simulink model "gm_smartCart4_1_work"  (R2016a)
settings: Solver=FixedStepDiscrete  StartTime=0.0  StopTime=100000  FixedStep=1  RelTol=1e-3
libraries: simulink x103, hdlsllib x73
(part 1 of 3)
settings Model: Creator=Admin  LastModifiedBy=Admin
settings OptimizationCC: BlockReduction=off  ConditionallyExecuteInputs=off  DefaultParameterBehavior=Inlined
settings DebuggingCC: AlgebraicLoopMsg=error  InheritedTsInSrcMsg=none
settings HardwareCC: ProdBitPerPointer=32  ProdLargestAtomicFloat=None  ProdIntDivRoundTo=Undefined  ProdEndianess=Unspecified  ProdWordSize=32  ProdHWDeviceType=ASIC/FPGA->ASIC/FPGA  ProdEqTarget=off

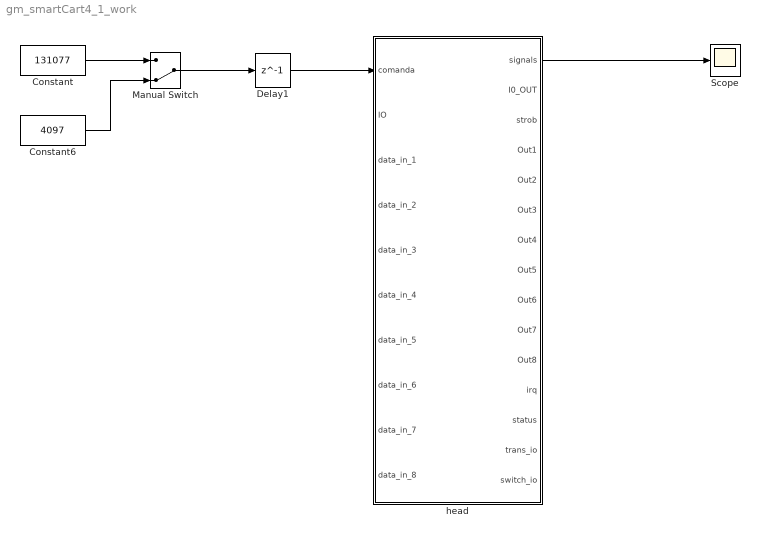
== system gm_smartCart4_1_work ==
  Constant : Constant  Value=131077  OutDataTypeStr=uint32  SampleTime=-1
  Constant6 : Constant  Value=4097  OutDataTypeStr=uint32  SampleTime=-1
  Delay1 : Delay  DelayLength=1  InitialCondition=0
  Manual Switch : ManualSwitch  CurrentSetting=0
  Scope : Scope
  head : Subsystem  TreatAsAtomicUnit=on
  wires:
  head/1(signals) -> Scope/1
  Delay1/1 -> head/1(comanda)
  Manual Switch/1 -> Delay1/1
  Constant6/1 -> Manual Switch/2
  Constant/1 -> Manual Switch/1

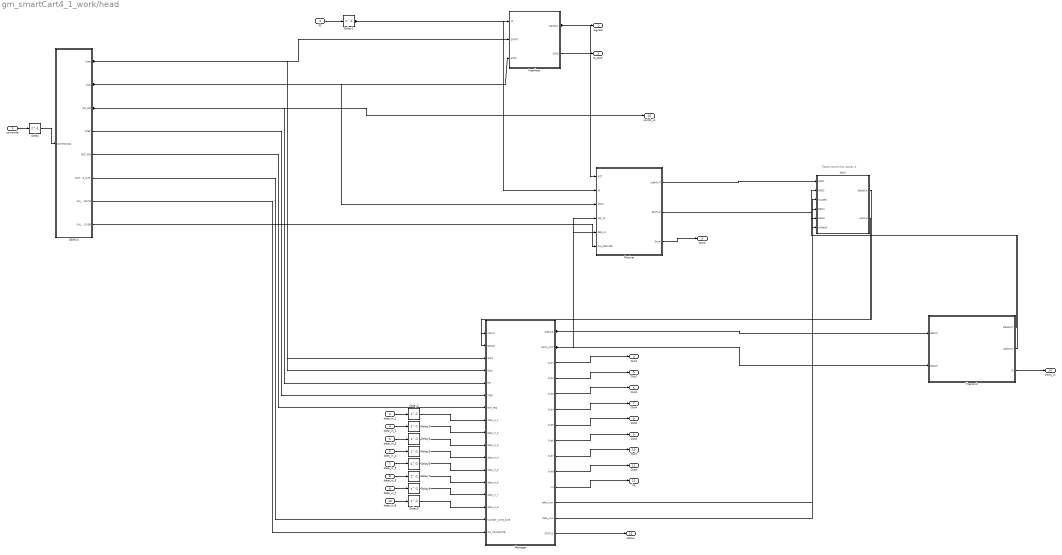
== system gm_smartCart4_1_work/head ==
  note: Переключатель адрес 4
  comanda : Inport  OutDataTypeStr=uint32  SampleTime=1
  IO : Inport  Port=2  OutDataTypeStr=boolean
  data_in_1 : Inport  Port=3  OutDataTypeStr=uint32
  data_in_2 : Inport  Port=4  OutDataTypeStr=uint32
  data_in_3 : Inport  Port=5  OutDataTypeStr=uint32
  data_in_4 : Inport  Port=6  OutDataTypeStr=uint32
  data_in_5 : Inport  Port=7  OutDataTypeStr=uint32
  data_in_6 : Inport  Port=8  OutDataTypeStr=uint32
  data_in_7 : Inport  Port=9  OutDataTypeStr=uint32
  data_in_8 : Inport  Port=10  OutDataTypeStr=uint32
  DEMUX : Subsystem
  Delay{,1..9} (10 alike) : Delay  DelayLength=1  InitialCondition=0
  Interface : Subsystem
  MUX : Subsystem
  Manager : Subsystem
  Reciver : Subsystem
  Transmit : Subsystem
  signals : Outport  OutDataTypeStr=fixdt(1,4,0)
  I0_OUT : Outport  Port=2  OutDataTypeStr=boolean
  strob : Outport  Port=3  OutDataTypeStr=boolean
  Out1 : Outport  Port=4  OutDataTypeStr=uint8
  Out2 : Outport  Port=5  OutDataTypeStr=uint8
  Out3 : Outport  Port=6  OutDataTypeStr=uint8
  Out4 : Outport  Port=7  OutDataTypeStr=uint8
  Out5 : Outport  Port=8  OutDataTypeStr=uint8
  Out6 : Outport  Port=9  OutDataTypeStr=uint8
  Out7 : Outport  Port=10  OutDataTypeStr=uint8
  Out8 : Outport  Port=11  OutDataTypeStr=uint8
  irq : Outport  Port=12  OutDataTypeStr=boolean
  status : Outport  Port=13  OutDataTypeStr=uint32
  trans_io : Outport  Port=14  OutDataTypeStr=boolean
  switch_io : Outport  Port=15  OutDataTypeStr=boolean
  wires:
  comanda/1 -> Delay/1
  IO/1 -> Delay1/1
  data_in_1/1 -> Delay2/1
  data_in_2/1 -> Delay3/1
  data_in_3/1 -> Delay4/1
  data_in_4/1 -> Delay5/1
  data_in_5/1 -> Delay6/1
  data_in_6/1 -> Delay7/1
  data_in_7/1 -> Delay8/1
  data_in_8/1 -> Delay9/1
  DEMUX/1(start) -> Interface/2(START), Manager/3(Start)
  DEMUX/2(stop) -> Interface/3(STOP), Reciver/3(STOP), Manager/4(Stop)
  DEMUX/3(RD_WR) -> Manager/5(RD), switch_io/1
  DEMUX/4(STEP) -> Manager/6(STEP)
  DEMUX/5(RST_IRQ) -> Manager/7(RST_IRQ)
  DEMUX/6(Number_write_byte) -> Manager/16(Number_write_byte)
  DEMUX/7(ON_TRANSMITE) -> Manager/17(ON_TRANSMITE)
  DEMUX/8(ON_RECIVER) -> Reciver/6(ON_RECIVER)
  Delay/1 -> DEMUX/1(COMMANDA)
  Delay1/1 -> Reciver/2(IO), Interface/1(IO)
  Delay2/1 -> Manager/8(data_in_1)
  Delay3/1 -> Manager/9(data_in_2)
  Delay4/1 -> Manager/10(data_in_3)
  Delay5/1 -> Manager/11(data_in_4)
  Delay6/1 -> Manager/12(data_in_5)
  Delay7/1 -> Manager/13(data_in_6)
  Delay8/1 -> Manager/14(data_in_7)
  Delay9/1 -> Manager/15(data_in_8)
  Interface/1(signals2) -> Reciver/1(RST), signals/1
  Interface/2(Out3) -> I0_OUT/1
  MUX/1(DataOut) -> Manager/2(DataIN)
  MUX/2(AdrOut) -> Manager/1(AdrrIN)
  Manager/1(addrout) -> Transmit/1(addrIN), Reciver/4(adr_IN)
  Manager/2(DATA_OUT) -> Transmit/2(dataIN), Reciver/5(data_in)
  Manager/3(Out1) -> Out1/1
  Manager/4(Out2) -> Out2/1
  Manager/5(Out3) -> Out3/1
  Manager/6(Out4) -> Out4/1
  Manager/7(Out5) -> Out5/1
  Manager/8(Out6) -> Out6/1
  Manager/9(Out7) -> Out7/1
  Manager/10(Out8) -> Out8/1
  Manager/11(irq) -> irq/1
  Manager/12(addr_mux) -> MUX/3(mADR3)
  Manager/13(data_mux) -> MUX/6(mData3)
  Manager/14(STATUS) -> status/1
  Reciver/1(AddrOUT) -> MUX/1(ADR1)
  Reciver/2(STATUS) -> MUX/4(Data1)
  Reciver/3(Strob) -> strob/1
  Transmit/1(DataOUT) -> MUX/5(Data2)
  Transmit/2(addrOUT) -> MUX/2(ADR2)
  Transmit/3(IO) -> trans_io/1

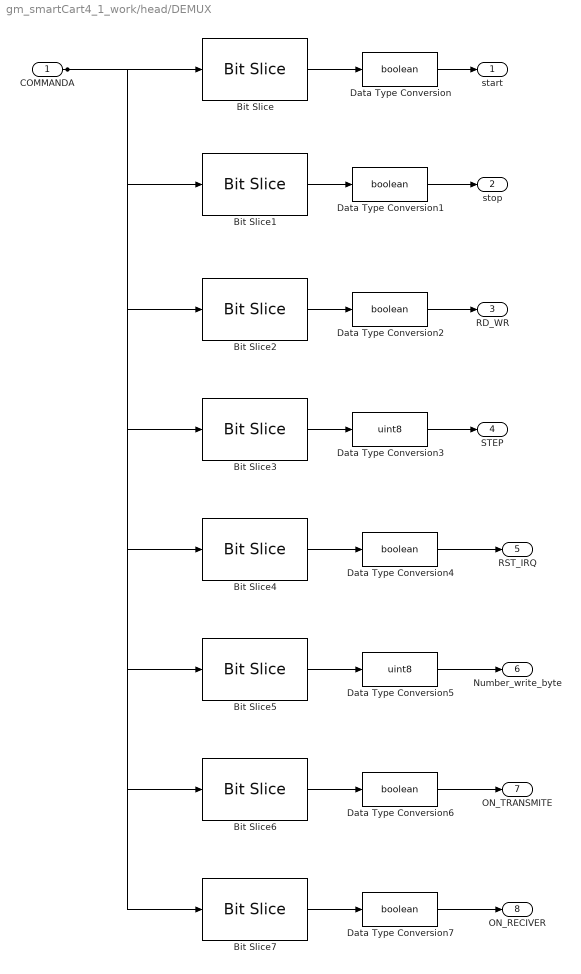
== system gm_smartCart4_1_work/head/DEMUX ==
  COMMANDA : Inport  OutDataTypeStr=uint32  SampleTime=1
  Bit Slice : hdlsllib/HDL Operations/Bit Slice  lidx=0  ridx=0
  Bit Slice1 : hdlsllib/HDL Operations/Bit Slice  lidx=1  ridx=1
  Bit Slice2 : hdlsllib/HDL Operations/Bit Slice  lidx=2  ridx=2
  Bit Slice3 : hdlsllib/HDL Operations/Bit Slice  lidx=11  ridx=3
  Bit Slice4 : hdlsllib/HDL Operations/Bit Slice  lidx=12  ridx=12
  Bit Slice5 : hdlsllib/HDL Operations/Bit Slice  lidx=15  ridx=13
  Bit Slice6 : hdlsllib/HDL Operations/Bit Slice  lidx=16  ridx=16
  Bit Slice7 : hdlsllib/HDL Operations/Bit Slice  lidx=17  ridx=17
  Data Type Conversion{,1..2,4,6..7} (6 alike) : DataTypeConversion  OutDataTypeStr=boolean
  Data Type Conversion3 : DataTypeConversion  OutDataTypeStr=uint8
  Data Type Conversion5 : DataTypeConversion  OutDataTypeStr=uint8
  start : Outport
  stop : Outport  Port=2
  RD_WR : Outport  Port=3
  STEP : Outport  Port=4  OutDataTypeStr=uint8
  RST_IRQ : Outport  Port=5
  Number_write_byte : Outport  Port=6  OutDataTypeStr=uint8
  ON_TRANSMITE : Outport  Port=7  OutDataTypeStr=boolean
  ON_RECIVER : Outport  Port=8  OutDataTypeStr=boolean
  wires:
  COMMANDA/1 -> Bit Slice7/1, Bit Slice6/1, Bit Slice5/1, Bit Slice4/1, Bit Slice3/1, Bit Slice2/1, Bit Slice1/1, Bit Slice/1
  Bit Slice/1 -> Data Type Conversion/1
  Bit Slice1/1 -> Data Type Conversion1/1
  Bit Slice2/1 -> Data Type Conversion2/1
  Bit Slice3/1 -> Data Type Conversion3/1
  Bit Slice4/1 -> Data Type Conversion4/1
  Bit Slice5/1 -> Data Type Conversion5/1
  Bit Slice6/1 -> Data Type Conversion6/1
  Bit Slice7/1 -> Data Type Conversion7/1
  Data Type Conversion/1 -> start/1
  Data Type Conversion1/1 -> stop/1
  Data Type Conversion2/1 -> RD_WR/1
  Data Type Conversion3/1 -> STEP/1
  Data Type Conversion4/1 -> RST_IRQ/1
  Data Type Conversion5/1 -> Number_write_byte/1
  Data Type Conversion6/1 -> ON_TRANSMITE/1
  Data Type Conversion7/1 -> ON_RECIVER/1

== system gm_smartCart4_1_work/head/Interface ==
  IO : Inport  OutDataTypeStr=boolean  SampleTime=1
  START : Inport  Port=2  OutDataTypeStr=boolean  SampleTime=1
  STOP : Inport  Port=3  OutDataTypeStr=boolean  SampleTime=1
  ColdStart : Subsystem
  ColdStop2 : Subsystem
  Head2 : Subsystem
  MUX2 : Subsystem
  Swith_signal2 : Subsystem
  signals2 : Outport  OutDataTypeStr=fixdt(1,4,0)  InitialOutput=0
  Out3 : Outport  Port=2  OutDataTypeStr=boolean  InitialOutput=0
  wires:
  IO/1 -> Out3/1, ColdStart/1(Reqest)
  START/1 -> Head2/3(START)
  STOP/1 -> Head2/4(STOP)
  ColdStart/1(DataOUT) -> MUX2/5(DAT_ST1)
  ColdStart/2(Signal) -> MUX2/2(DATA_0)
  ColdStart/3(ADR_OUT) -> MUX2/4(ADR_ST)
  ColdStop2/1(DataOUT) -> MUX2/7(DAT_STOP)
  ColdStop2/2(Signal) -> MUX2/3(DATA_1)
  ColdStop2/3(ADR_OUT) -> MUX2/6(ADR_STOP)
  Head2/1(AdrOut) -> Swith_signal2/1(Adr), ColdStart/2(Addr), ColdStop2/1(Addr)
  Head2/2(DataOut) -> Swith_signal2/2(Data), ColdStart/3(Data), ColdStop2/2(Data)
  MUX2/1(Signals) -> signals2/1
  MUX2/2(ADR_OUT) -> Head2/1(ADR_IN)
  MUX2/3(DATA_OUT1) -> Head2/2(DataIN)
  Swith_signal2/1(OutAddr) -> MUX2/1(ADR)

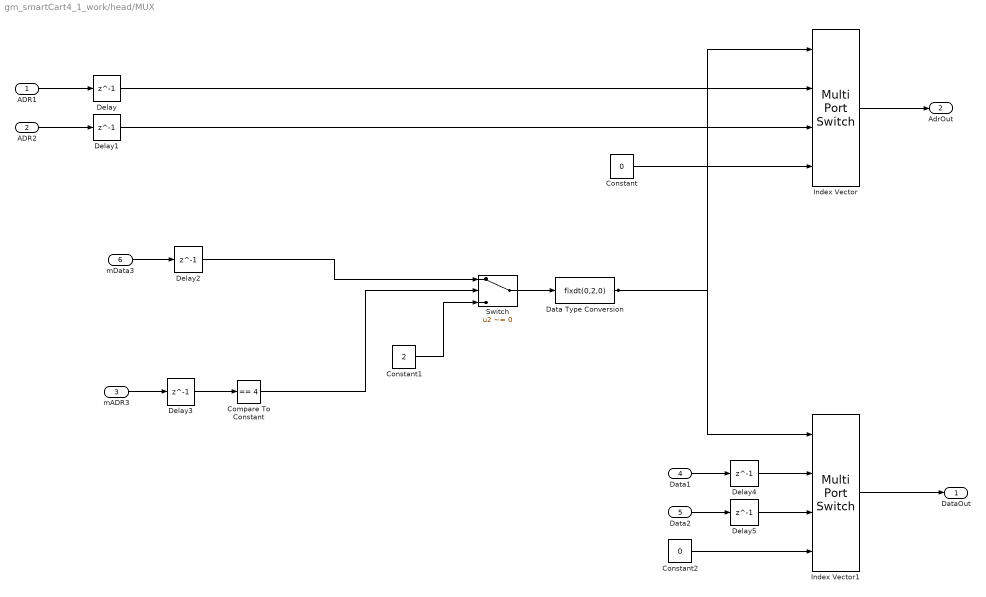
== system gm_smartCart4_1_work/head/MUX ==
  ADR1 : Inport  OutDataTypeStr=uint8  SampleTime=1
  ADR2 : Inport  Port=2  OutDataTypeStr=uint8  SampleTime=1
  mADR3 : Inport  Port=3  OutDataTypeStr=uint8  SampleTime=1
  Data1 : Inport  Port=4  OutDataTypeStr=uint32  SampleTime=1
  Data2 : Inport  Port=5  OutDataTypeStr=uint32  SampleTime=1
  mData3 : Inport  Port=6  OutDataTypeStr=uint32  SampleTime=1
  Compare To Constant : simulink/Logic and Bit Operations/Compare To Constant  relop===  const=4  OutDataTypeStr=boolean
  Constant : Constant  Value=0  OutDataTypeStr=uint8
  Constant1 : Constant  Value=2  OutDataTypeStr=uint32
  Constant2 : Constant  Value=0  OutDataTypeStr=uint32
  Data Type Conversion : DataTypeConversion  OutDataTypeStr=fixdt(0,2,0)
  Delay{,1..5} (6 alike) : Delay  DelayLength=1  InitialCondition=0
  Index Vector : MultiPortSwitch  DataPortOrder=Zero-based contiguous  zeroidx=on
  Index Vector1 : MultiPortSwitch  DataPortOrder=Zero-based contiguous  zeroidx=on
  Switch : Switch  Criteria=u2 ~= 0
  DataOut : Outport  OutDataTypeStr=uint32
  AdrOut : Outport  Port=2  OutDataTypeStr=uint8
  wires:
  ADR1/1 -> Delay/1
  ADR2/1 -> Delay1/1
  mADR3/1 -> Delay3/1
  Data1/1 -> Delay4/1
  Data2/1 -> Delay5/1
  mData3/1 -> Delay2/1
  Compare To Constant/1 -> Switch/2
  Constant/1 -> Index Vector/4
  Constant1/1 -> Switch/3
  Constant2/1 -> Index Vector1/4
  Data Type Conversion/1 -> Index Vector1/1, Index Vector/1
  Delay/1 -> Index Vector/2
  Delay1/1 -> Index Vector/3
  Delay2/1 -> Switch/1
  Delay3/1 -> Compare To Constant/1
  Delay4/1 -> Index Vector1/2
  Delay5/1 -> Index Vector1/3
  Index Vector/1 -> AdrOut/1
  Index Vector1/1 -> DataOut/1
  Switch/1 -> Data Type Conversion/1

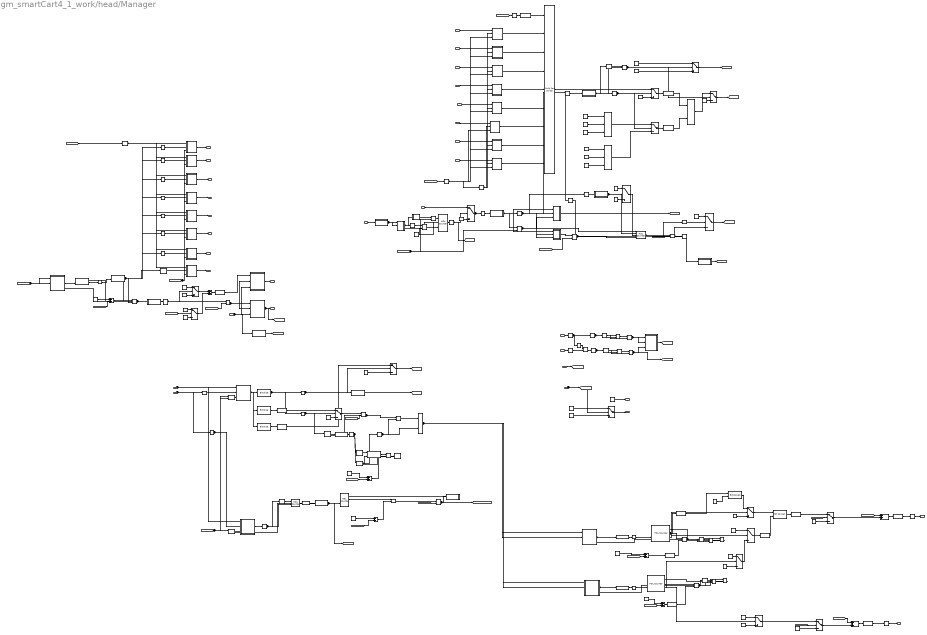
== system gm_smartCart4_1_work/head/Manager ==
  note: Схема управления передатчиком
  note: Схема управления приёмника
  note: Схема включения и выключения
  note: Схема синхр
  note: Схема декодирования команд
  note: Декодер команд
  AdrrIN : Inport  OutDataTypeStr=uint8  SampleTime=1
  DataIN : Inport  Port=2  OutDataTypeStr=uint32  SampleTime=1
  Start : Inport  Port=3  OutDataTypeStr=boolean  SampleTime=1
  Stop : Inport  Port=4  OutDataTypeStr=boolean  SampleTime=1
  RD : Inport  Port=5  OutDataTypeStr=boolean  SampleTime=1
  STEP : Inport  Port=6  OutDataTypeStr=uint8  SampleTime=1
  RST_IRQ : Inport  Port=7  OutDataTypeStr=boolean  SampleTime=1
  data_in_1 : Inport  Port=8  OutDataTypeStr=uint32  SampleTime=1
  data_in_2 : Inport  Port=9  OutDataTypeStr=uint32  SampleTime=1
  data_in_3 : Inport  Port=10  OutDataTypeStr=uint32  SampleTime=1
  data_in_4 : Inport  Port=11  OutDataTypeStr=uint32  SampleTime=1
  data_in_5 : Inport  Port=12  OutDataTypeStr=uint32  SampleTime=1
  data_in_6 : Inport  Port=13  OutDataTypeStr=uint32  SampleTime=1
  data_in_7 : Inport  Port=14  OutDataTypeStr=uint32  SampleTime=1
  data_in_8 : Inport  Port=15  OutDataTypeStr=uint32  SampleTime=1
  Number_write_byte : Inport  Port=16  OutDataTypeStr=uint8  SampleTime=1
  ON_TRANSMITE : Inport  Port=17  OutDataTypeStr=boolean  SampleTime=1
  Add{,1..7} (8 alike) : Sum
  Bit Concat : hdlsllib/HDL Operations/Bit Concat  numInputs=2
  Bit Concat1 : hdlsllib/HDL Operations/Bit Concat  numInputs=2
  Bit Concat2 : hdlsllib/HDL Operations/Bit Concat  numInputs=3
  Bit Concat3 : hdlsllib/HDL Operations/Bit Concat  numInputs=3
  Bit Concat4 : hdlsllib/HDL Operations/Bit Concat  numInputs=2
  Bit Slice3 : hdlsllib/HDL Operations/Bit Slice  lidx=1  ridx=0
  Bit Slice4 : hdlsllib/HDL Operations/Bit Slice  lidx=9  ridx=2
  Bit Slice5 : hdlsllib/HDL Operations/Bit Slice  lidx=17  ridx=10
  Compare To Constant{,1..6,10,12,20..21} (11 alike) : simulink/Logic and Bit Operations/Compare To Constant  relop===  const=1  OutDataTypeStr=boolean
  Compare To Constant11 : simulink/Logic and Bit Operations/Compare To Constant  relop===  const=4  OutDataTypeStr=boolean
  Compare To Constant13 : simulink/Logic and Bit Operations/Compare To Constant  relop===  const=2  OutDataTypeStr=boolean
  Compare To Constant14 : simulink/Logic and Bit Operations/Compare To Constant  relop===  const=5  OutDataTypeStr=boolean
  Compare To Constant15 : simulink/Logic and Bit Operations/Compare To Constant  relop===  const=6  OutDataTypeStr=boolean
  Compare To Constant16 : simulink/Logic and Bit Operations/Compare To Constant  relop===  const=7  OutDataTypeStr=boolean
  Compare To Constant17 : simulink/Logic and Bit Operations/Compare To Constant  relop===  const=8  OutDataTypeStr=boolean
  Compare To Constant18 : simulink/Logic and Bit Operations/Compare To Constant  relop=~=  const=255  OutDataTypeStr=boolean
  Compare To Constant19 : simulink/Logic and Bit Operations/Compare To Constant  relop===  const=100  OutDataTypeStr=boolean
  Compare To Constant22 : simulink/Logic and Bit Operations/Compare To Constant  relop===  const=5208*2  OutDataTypeStr=boolean
  Compare To Constant23 : simulink/Logic and Bit Operations/Compare To Constant  relop===  const=255  OutDataTypeStr=boolean
  Compare To Constant24 : simulink/Logic and Bit Operations/Compare To Constant  relop===  const=0  OutDataTypeStr=boolean
  Compare To Constant7 : simulink/Logic and Bit Operations/Compare To Constant  relop===  const=2  OutDataTypeStr=boolean
  Compare To Constant8 : simulink/Logic and Bit Operations/Compare To Constant  relop===  const=3  OutDataTypeStr=boolean
  Compare To Constant9 : simulink/Logic and Bit Operations/Compare To Constant  relop===  const=2  OutDataTypeStr=boolean
  Constant{,2,12..15,23,25,28,36} (10 alike) : Constant  Value=0  OutDataTypeStr=uint8  SampleTime=-1
  Constant{1,3,7,10,24} (5 alike) : Constant  OutDataTypeStr=uint8  SampleTime=-1
  Constant11 : Constant  Value=4  OutDataTypeStr=uint8  SampleTime=-1
  Constant{5,16,18,26} (4 alike) : Constant  OutDataTypeStr=boolean  SampleTime=-1
  Constant{6,17,22,31,33..34} (6 alike) : Constant  Value=0  OutDataTypeStr=uint32  SampleTime=-1
  Constant19 : Constant  Value=0  OutDataTypeStr=boolean  SampleTime=-1
  Constant20 : Constant  Value=0  OutDataTypeStr=boolean  SampleTime=-1
  Constant21 : Constant  Value=0  OutDataTypeStr=boolean  SampleTime=-1
  Constant27 : Constant  Value=2  OutDataTypeStr=uint8  SampleTime=-1
  Constant29 : Constant  Value=255  OutDataTypeStr=uint8  SampleTime=-1
  Constant30 : Constant  OutDataTypeStr=uint32  SampleTime=-1
  Constant32 : Constant  Value=2  OutDataTypeStr=uint32  SampleTime=-1
  Constant35 : Constant  Value=255  OutDataTypeStr=uint8  SampleTime=-1
  Constant4 : Constant  Value=2  OutDataTypeStr=uint8  SampleTime=-1
  Constant8 : Constant  OutDataTypeStr=uint32  SampleTime=-1
  Constant9 : Constant  Value=2  OutDataTypeStr=uint8  SampleTime=-1
  Data Type Conversion{,3..4,7..8} (5 alike) : DataTypeConversion  OutDataTypeStr=uint8
  Data Type Conversion1 : DataTypeConversion  OutDataTypeStr=uint32
  Data Type Conversion10 : DataTypeConversion  OutDataTypeStr=fixdt(0,2,0)
  Data Type Conversion11 : DataTypeConversion  OutDataTypeStr=fixdt(0,3,0)
  Data Type Conversion12 : DataTypeConversion  OutDataTypeStr=uint32
  Data Type Conversion2 : DataTypeConversion  OutDataTypeStr=fixdt(0,3,0)
  Data Type Conversion5 : DataTypeConversion  OutDataTypeStr=uint32
  Data Type Conversion6 : DataTypeConversion  OutDataTypeStr=fixdt(0,4,0)
  Data Type Conversion9 : DataTypeConversion  OutDataTypeStr=fixdt(0,4,0)
  Delay{,1..3,5..16} (16 alike) : Delay  DelayLength=1  InitialCondition=0
  Delay4 : Delay  DelayLength=3  InitialCondition=0
  HDL Counter1 : hdlsllib/HDL Operations/HDL Counter  CountType=Free running  CountInit=0  CountStep=1  CountMax=25  CountFromType=Initial value  CountFrom=0  CountResetPort=on  CountLoadPort=off  CountEnbPort=on  CountDirPort=off  CountDataType=Unsigned  CountWordLen=4  CountFracLen=0  CountSampTime=1
  HDL Counter10 : hdlsllib/HDL Operations/HDL Counter  CountType=Free running  CountInit=255  CountStep=1  CountMax=25  CountFromType=Initial value  CountFrom=255  CountResetPort=on  CountLoadPort=off  CountEnbPort=on  CountDirPort=off  CountDataType=Unsigned  CountWordLen=8  CountFracLen=0  CountSampTime=1
  HDL Counter11 : hdlsllib/HDL Operations/HDL Counter  CountType=Count limited  CountInit=0  CountStep=1  CountMax=5208*2  CountFromType=Initial value  CountFrom=0  CountResetPort=on  CountLoadPort=off  CountEnbPort=on  CountDirPort=off  CountDataType=Unsigned  CountWordLen=14  CountFracLen=0  CountSampTime=1
  HDL Counter12 : hdlsllib/HDL Operations/HDL Counter  CountType=Count limited  CountInit=0  CountStep=1  CountMax=100  CountFromType=Initial value  CountFrom=0  CountResetPort=on  CountLoadPort=off  CountEnbPort=on  CountDirPort=off  CountDataType=Unsigned  CountWordLen=8  CountFracLen=0  CountSampTime=1
  HDL Counter2 : hdlsllib/HDL Operations/HDL Counter  CountType=Free running  CountInit=0  CountStep=1  CountMax=25  CountFromType=Initial value  CountFrom=0  CountResetPort=on  CountLoadPort=off  CountEnbPort=on  CountDirPort=off  CountDataType=Unsigned  CountWordLen=4  CountFracLen=0  CountSampTime=1
  HDL Counter3 : hdlsllib/HDL Operations/HDL Counter  CountType=Free running  CountInit=0  CountStep=1  CountMax=25  CountFromType=Initial value  CountFrom=0  CountResetPort=on  CountLoadPort=off  CountEnbPort=on  CountDirPort=off  CountDataType=Unsigned  CountWordLen=8  CountFracLen=0  CountSampTime=1
  HDL Counter4 : hdlsllib/HDL Operations/HDL Counter  CountType=Free running  CountInit=0  CountStep=1  CountMax=25  CountFromType=Initial value  CountFrom=0  CountResetPort=on  CountLoadPort=off  CountEnbPort=on  CountDirPort=off  CountDataType=Unsigned  CountWordLen=4  CountFracLen=0  CountSampTime=1
  HDL Counter5 : hdlsllib/HDL Operations/HDL Counter  CountType=Free running  CountInit=0  CountStep=1  CountMax=25  CountFromType=Initial value  CountFrom=0  CountResetPort=off  CountLoadPort=off  CountEnbPort=on  CountDirPort=off  CountDataType=Unsigned  CountWordLen=1  CountFracLen=0  CountSampTime=1
  HDL Counter6 : hdlsllib/HDL Operations/HDL Counter  CountType=Free running  CountInit=0  CountStep=1  CountMax=25  CountFromType=Initial value  CountFrom=0  CountResetPort=off  CountLoadPort=off  CountEnbPort=on  CountDirPort=off  CountDataType=Unsigned  CountWordLen=1  CountFracLen=0  CountSampTime=1
  HDL Counter7 : hdlsllib/HDL Operations/HDL Counter  CountType=Free running  CountInit=0  CountStep=1  CountMax=25  CountFromType=Initial value  CountFrom=0  CountResetPort=off  CountLoadPort=off  CountEnbPort=on  CountDirPort=off  CountDataType=Unsigned  CountWordLen=1  CountFracLen=0  CountSampTime=1
  HDL Counter8 : hdlsllib/HDL Operations/HDL Counter  CountType=Free running  CountInit=0  CountStep=1  CountMax=25  CountFromType=Initial value  CountFrom=0  CountResetPort=on  CountLoadPort=off  CountEnbPort=on  CountDirPort=off  CountDataType=Unsigned  CountWordLen=1  CountFracLen=0  CountSampTime=1
  HDL Counter9 : hdlsllib/HDL Operations/HDL Counter  CountType=Free running  CountInit=0  CountStep=1  CountMax=25  CountFromType=Initial value  CountFrom=0  CountResetPort=on  CountLoadPort=on  CountEnbPort=on  CountDirPort=off  CountDataType=Unsigned  CountWordLen=8  CountFracLen=0  CountSampTime=1
  Index Vector : MultiPortSwitch  DataPortOrder=Zero-based contiguous  Inputs=8  zeroidx=on
  Logical Operator{,2,7,10} (4 alike) : Logic  Operator=XOR  AllPortsSameDT=off  OutDataTypeStr=boolean
  Logical Operator{1,3..4,6,8..9,12,15,17,19,26} (11 alike) : Logic  AllPortsSameDT=off  OutDataTypeStr=boolean
  Logical Operator{5,11,16,18,21,25} (6 alike) : Logic  Operator=NOT  AllPortsSameDT=off  OutDataTypeStr=boolean
  Logical Operator{13..14,20,22..24,28} (7 alike) : Logic  Operator=OR  AllPortsSameDT=off  OutDataTypeStr=boolean
  Logical Operator27 : Logic  Inputs=3  AllPortsSameDT=off  OutDataTypeStr=boolean
  Logical Operator29 : Logic  Operator=NOT  Inputs=3  AllPortsSameDT=off  OutDataTypeStr=boolean
  Relational Operator{,1..4,7..8} (7 alike) : RelationalOperator  Operator===  OutDataTypeStr=boolean
  Switch{1..18} (18 alike) : Switch  Criteria=u2 ~= 0
  Unit Delay Enabled Resettable : Subsystem
  Unit Delay Enabled Resettable1 : Subsystem
  Unit Delay Enabled Resettable10 : Subsystem
  Unit Delay Enabled Resettable11 : Subsystem
  Unit Delay Enabled Resettable12 : Subsystem
  Unit Delay Enabled Resettable13 : Subsystem
  Unit Delay Enabled Resettable14 : Subsystem
  Unit Delay Enabled Resettable15 : Subsystem
  Unit Delay Enabled Resettable16 : Subsystem
  Unit Delay Enabled Resettable17 : Subsystem
  Unit Delay Enabled Resettable18 : Subsystem
  Unit Delay Enabled Resettable19 : Subsystem
  Unit Delay Enabled Resettable2 : Subsystem
  Unit Delay Enabled Resettable20 : Subsystem
  Unit Delay Enabled Resettable21 : Subsystem
  Unit Delay Enabled Resettable22 : Subsystem
  Unit Delay Enabled Resettable23 : Subsystem
  Unit Delay Enabled Resettable24 : Subsystem
  Unit Delay Enabled Resettable26 : Subsystem
  Unit Delay Enabled Resettable28 : Subsystem
  Unit Delay Enabled Resettable3 : Subsystem
  Unit Delay Enabled Resettable4 : Subsystem
  Unit Delay Enabled Resettable5 : Subsystem
  Unit Delay Enabled Resettable6 : Subsystem
  Unit Delay Enabled Resettable7 : Subsystem
  Unit Delay Enabled Resettable8 : Subsystem
  Unit Delay Enabled Resettable9 : Subsystem
  signal_edg : Subsystem
  signal_edg1 : Subsystem
  signal_edg10 : Subsystem
  signal_edg2 : Subsystem
  signal_edg3 : Subsystem
  signal_edg4 : Subsystem
  signal_edg5 : Subsystem
  signal_edg6 : Subsystem
  signal_edg7 : Subsystem
  signal_edg8 : Subsystem
  signal_edg9 : Subsystem
  addrout : Outport  OutDataTypeStr=uint8
  DATA_OUT : Outport  Port=2  OutDataTypeStr=uint32
  Out1 : Outport  Port=3  OutDataTypeStr=uint8
  Out2 : Outport  Port=4  OutDataTypeStr=uint8
  Out3 : Outport  Port=5  OutDataTypeStr=uint8
  Out4 : Outport  Port=6  OutDataTypeStr=uint8
  Out5 : Outport  Port=7  OutDataTypeStr=uint8
  Out6 : Outport  Port=8  OutDataTypeStr=uint8
  Out7 : Outport  Port=9  OutDataTypeStr=uint8
  Out8 : Outport  Port=10  OutDataTypeStr=uint8
  irq : Outport  Port=11  OutDataTypeStr=boolean
  addr_mux : Outport  Port=12  OutDataTypeStr=uint8
  data_mux : Outport  Port=13  OutDataTypeStr=uint32
  STATUS : Outport  Port=14  OutDataTypeStr=uint32
  wires:
  AdrrIN/1 -> Compare To Constant13/1, Compare To Constant12/1
  DataIN/1 -> Unit Delay Enabled Resettable2/1(data_in), Unit Delay Enabled Resettable1/1(data_in)
  Start/1 -> Delay13/1
  Stop/1 -> Delay14/1
  RD/1 -> Switch5/2, [INST_WORK]
  STEP/1 -> [INST_WORK_VAL]
  RST_IRQ/1 -> Unit Delay Enabled Resettable26/3(Reset), Unit Delay Enabled Resettable14/3(Reset), signal_edg10/1(In1)
  data_in_1/1 -> Unit Delay Enabled Resettable17/1(data_in)
  data_in_2/1 -> Unit Delay Enabled Resettable18/1(data_in)
  data_in_3/1 -> Unit Delay Enabled Resettable19/1(data_in)
  data_in_4/1 -> Unit Delay Enabled Resettable20/1(data_in)
  data_in_5/1 -> Unit Delay Enabled Resettable21/1(data_in)
  data_in_6/1 -> Unit Delay Enabled Resettable22/1(data_in)
  data_in_7/1 -> Unit Delay Enabled Resettable23/1(data_in)
  data_in_8/1 -> Unit Delay Enabled Resettable24/1(data_in)
  Number_write_byte/1 -> Switch17/1
  ON_TRANSMITE/1 -> signal_edg7/1(In1)
  Add/1 -> Data Type Conversion6/1
  Add1/1 -> Data Type Conversion4/1
  Add2/1 -> Data Type Conversion5/1
  Add3/1 -> Data Type Conversion9/1
  Add4/1 -> Relational Operator3/1
  Add5/1 -> Relational Operator4/2
  Add6/1 -> Data Type Conversion12/1
  Add7/1 -> Relational Operator7/2
  Bit Concat/1 -> Data Type Conversion1/1
  Bit Concat1/1 -> Switch2/1
  Bit Concat2/1 -> Switch7/1
  Bit Concat3/1 -> Switch7/3
  Bit Concat4/1 -> Switch16/1
  Bit Slice3/1 -> Compare To Constant9/1, Compare To Constant10/1
  Bit Slice4/1 -> Data Type Conversion7/1
  Bit Slice5/1 -> Data Type Conversion8/1
  Compare To Constant/1 -> Logical Operator1/2, Logical Operator/2, Delay/1
  Compare To Constant1/1 -> Logical Operator3/2, Logical Operator2/2, Delay1/1
  Compare To Constant10/1 -> Switch10/2, Logical Operator19/1
  Compare To Constant11/1 -> Unit Delay Enabled Resettable9/2(Enb)
  Compare To Constant12/1 -> Unit Delay Enabled Resettable1/2(Enb)
  Compare To Constant13/1 -> Logical Operator14/2, Unit Delay Enabled Resettable2/2(Enb)
  Compare To Constant14/1 -> Unit Delay Enabled Resettable10/2(Enb)
  Compare To Constant15/1 -> Unit Delay Enabled Resettable11/2(Enb)
  Compare To Constant16/1 -> Unit Delay Enabled Resettable12/2(Enb)
  Compare To Constant17/1 -> Unit Delay Enabled Resettable13/2(Enb)
  Compare To Constant18/1 -> signal_edg1/1(In1)
  Compare To Constant19/1 -> Switch17/2, Logical Operator16/1, Unit Delay Enabled Resettable16/3(Reset), [ON_TRANS]
  Compare To Constant2/1 -> HDL Counter3/2
  Compare To Constant20/1 -> Logical Operator21/1, Unit Delay Enabled Resettable24/3(Reset), Unit Delay Enabled Resettable23/3(Reset), Unit Delay Enabled Resettable22/3(Reset), Unit Delay Enabled Resettable21/3(Reset), Unit Delay Enabled Resettable20/3(Reset), Unit Delay Enabled Resettable19/3(Reset), Unit Delay Enabled Resettable18/3(Reset), Unit Delay Enabled Resettable17/3(Reset)
  Compare To Constant21/1 -> Logical Operator25/1, HDL Counter11/2
  Compare To Constant22/1 -> signal_edg5/1(In1)
  Compare To Constant23/1 -> Switch4/2
  Compare To Constant24/1 -> signal_edg9/1(In1)
  Compare To Constant3/1 -> Logical Operator12/1, Logical Operator11/1
  Compare To Constant4/1 -> HDL Counter1/2
  Compare To Constant5/1 -> HDL Counter2/2
  Compare To Constant6/1 -> Unit Delay Enabled Resettable6/2(Enb)
  Compare To Constant7/1 -> Unit Delay Enabled Resettable7/2(Enb)
  Compare To Constant8/1 -> Unit Delay Enabled Resettable8/2(Enb)
  Compare To Constant9/1 -> Switch9/2, signal_edg/1(In1)
  Constant/1 -> Switch2/3
  Constant1/1 -> Switch1/1
  Constant10/1 -> Add5/1
  Constant11/1 -> addr_mux/1
  Constant12/1 -> Add7/1
  Constant13/1 -> Switch4/1
  Constant14/1 -> Switch9/3
  Constant15/1 -> Switch10/3
  Constant16/1 -> Bit Concat2/3
  Constant17/1 -> Switch6/3
  Constant18/1 -> Bit Concat2/2
  Constant19/1 -> Bit Concat2/1
  Constant2/1 -> Switch1/3
  Constant20/1 -> Bit Concat3/3
  Constant21/1 -> Bit Concat3/2
  Constant22/1 -> Switch12/3
  Constant23/1 -> Switch13/3
  Constant24/1 -> Add3/1
  Constant25/1 -> Switch14/3
  Constant26/1 -> Bit Concat3/1
  Constant27/1 -> Switch8/1
  Constant28/1 -> Switch8/3
  Constant29/1 -> Switch18/1
  Constant3/1 -> Switch14/1
  Constant30/1 -> Switch11/1
  Constant31/1 -> Switch11/3
  Constant32/1 -> Switch15/1
  Constant33/1 -> Switch15/3
  Constant34/1 -> Switch16/3
  Constant35/1 -> Switch17/3
  Constant36/1 -> Switch18/3
  Constant4/1 -> Switch3/1
  Constant5/1 -> Bit Concat1/2
  Constant6/1 -> Switch5/1
  Constant7/1 -> Add4/1
  Constant8/1 -> Switch5/3
  Constant9/1 -> Add/1
  Data Type Conversion/1 -> Bit Concat1/1
  Data Type Conversion1/1 -> Switch12/1
  Data Type Conversion10/1 -> Bit Concat/2
  Data Type Conversion11/1 -> Bit Concat4/2
  Data Type Conversion12/1 -> Unit Delay Enabled Resettable26/1(data_in)
  Data Type Conversion2/1 -> Index Vector/1
  Data Type Conversion3/1 -> Bit Concat4/1
  Data Type Conversion4/1 -> Delay8/1
  Data Type Conversion5/1 -> Delay7/1
  Data Type Conversion6/1 -> Relational Operator2/2
  Data Type Conversion7/1 -> Switch10/1
  Data Type Conversion8/1 -> Switch9/1
  Data Type Conversion9/1 -> Relational Operator1/2
  Delay/1 -> Logical Operator/1
  Delay1/1 -> Logical Operator2/1
  Delay10/1 -> Switch7/2, Switch6/2
  Delay11/1 -> Logical Operator22/1
  Delay12/1 -> Data Type Conversion2/1
  Delay13/1 -> Logical Operator5/1, Compare To Constant/1
  Delay14/1 -> Logical Operator4/2
  Delay15/1 -> Logical Operator28/2
  Delay16/1 -> Logical Operator15/1
  Delay2/1 -> Logical Operator7/1
  Delay3/1 -> Logical Operator10/1
  Delay4/1 -> Unit Delay Enabled Resettable9/1(data_in), Unit Delay Enabled Resettable8/1(data_in), Unit Delay Enabled Resettable7/1(data_in), Unit Delay Enabled Resettable6/1(data_in), Unit Delay Enabled Resettable13/1(data_in), Unit Delay Enabled Resettable12/1(data_in), Unit Delay Enabled Resettable11/1(data_in), Unit Delay Enabled Resettable10/1(data_in)
  Delay5/1 -> Switch11/2, Logical Operator23/1
  Delay6/1 -> Logical Operator8/2, Logical Operator17/2
  Delay7/1 -> DATA_OUT/1
  Delay8/1 -> addrout/1
  Delay9/1 -> Logical Operator28/1, Unit Delay Enabled Resettable28/2(Enb), Unit Delay Enabled Resettable15/2(Enb)
  [INST_WORK_VAL] -> Relational Operator/2
  [INST_WORK_VAL] -> Add5/2
  [RST] -> Unit Delay Enabled Resettable9/3(Reset), Unit Delay Enabled Resettable8/3(Reset), Unit Delay Enabled Resettable7/3(Reset), Unit Delay Enabled Resettable6/3(Reset), Unit Delay Enabled Resettable13/3(Reset), Unit Delay Enabled Resettable12/3(Reset), Unit Delay Enabled Resettable11/3(Reset), Unit Delay Enabled Resettable10/3(Reset)
  [count_wr] -> Delay12/1
  [RST] -> Compare To Constant20/1
  [byte_done] -> Logical Operator27/3
  [ON_TRANS] -> Logical Operator26/2
  [rst_interrypt] -> Logical Operator24/2, Logical Operator20/2
  [addr_wr] -> Add1/1
  [data_wr] -> Add2/1
  [INST_WORK_VAL] -> Add/2
  [IRQ_TRANSMIT] -> Switch15/2
  [IRQ_TRANSMIT] -> Logical Operator23/2
  [num_wr_byt] -> Relational Operator8/2
  [num_wr_byt] -> Add7/2
  [RST] -> Logical Operator14/1, Logical Operator13/1
  [RD_BYTE] -> Unit Delay Enabled Resettable5/2(Enb), Unit Delay Enabled Resettable5/1(data_in)
  [INST_WORK] -> Switch12/2
  [INST_WORK] -> Switch13/2
  [INST_WORK_VAL] -> Add3/2
  [RD_BYTE_VAL] -> Delay4/1
  [INST_WORK_VAL] -> Add4/2
  HDL Counter1/1 -> Relational Operator1/1, Data Type Conversion/1
  HDL Counter10/1 -> Relational Operator7/1
  HDL Counter11/1 -> Compare To Constant22/1
  HDL Counter12/1 -> Compare To Constant19/1
  HDL Counter2/1 -> Relational Operator2/1
  HDL Counter3/1 -> Relational Operator3/2, Compare To Constant8/1, Compare To Constant7/1, Compare To Constant6/1, Compare To Constant17/1, Compare To Constant16/1, Compare To Constant15/1, Compare To Constant14/1, Compare To Constant11/1
  HDL Counter4/1 -> Relational Operator4/1
  HDL Counter5/1 -> Compare To Constant3/1
  HDL Counter6/1 -> Compare To Constant4/1
  HDL Counter7/1 -> Compare To Constant5/1
  HDL Counter8/1 -> Compare To Constant2/1
  HDL Counter9/1 -> Switch4/3, Relational Operator8/1, Compare To Constant23/1
  Index Vector/1 -> Switch6/1
  Logical Operator/1 -> Logical Operator1/1
  Logical Operator1/1 -> Unit Delay Enabled Resettable/2(Enb), Unit Delay Enabled Resettable/1(data_in)
  Logical Operator10/1 -> Logical Operator9/2
  Logical Operator11/1 -> HDL Counter4/1
  Logical Operator12/1 -> HDL Counter4/2, Delay6/1
  Logical Operator13/1 -> Unit Delay Enabled Resettable2/3(Reset)
  Logical Operator14/1 -> Unit Delay Enabled Resettable1/3(Reset)
  Logical Operator15/1 -> HDL Counter12/2
  Logical Operator16/1 -> Logical Operator15/2
  Logical Operator17/1 -> Logical Operator8/1
  Logical Operator18/1 -> Logical Operator12/2
  Logical Operator19/1 -> HDL Counter5/1
  Logical Operator2/1 -> Logical Operator3/1
  Logical Operator20/1 -> Unit Delay Enabled Resettable28/3(Reset), Unit Delay Enabled Resettable15/3(Reset), HDL Counter9/1
  Logical Operator21/1 -> Unit Delay Enabled Resettable24/2(Enb), Unit Delay Enabled Resettable23/2(Enb), Unit Delay Enabled Resettable22/2(Enb), Unit Delay Enabled Resettable21/2(Enb), Unit Delay Enabled Resettable20/2(Enb), Unit Delay Enabled Resettable19/2(Enb), Unit Delay Enabled Resettable18/2(Enb), Unit Delay Enabled Resettable17/2(Enb)
  Logical Operator22/1 -> Switch8/2, Switch16/2
  Logical Operator23/1 -> Unit Delay Enabled Resettable26/2(Enb), Unit Delay Enabled Resettable14/2(Enb), Unit Delay Enabled Resettable14/1(data_in)
  Logical Operator24/1 -> HDL Counter12/1
  Logical Operator25/1 -> HDL Counter11/1
  Logical Operator26/1 -> [IRQ_TRANSMIT], signal_edg3/1(In1)
  Logical Operator27/1 -> HDL Counter9/4, Delay15/1
  Logical Operator28/1 -> signal_edg2/1(In1)
  Logical Operator29/1 -> Logical Operator27/2
  Logical Operator3/1 -> Unit Delay Enabled Resettable/3(Reset), [RST]
  Logical Operator4/1 -> Compare To Constant1/1
  Logical Operator5/1 -> Logical Operator4/1
  Logical Operator6/1 -> HDL Counter1/1
  Logical Operator7/1 -> Logical Operator6/2
  Logical Operator8/1 -> Unit Delay Enabled Resettable4/2(Enb), Unit Delay Enabled Resettable4/1(data_in), Unit Delay Enabled Resettable3/2(Enb), Unit Delay Enabled Resettable3/1(data_in)
  Logical Operator9/1 -> HDL Counter2/1
  Relational Operator/1 -> Logical Operator19/2, Logical Operator17/1
  Relational Operator1/1 -> Logical Operator7/2, Logical Operator6/1, Unit Delay Enabled Resettable3/3(Reset), Delay2/1
  Relational Operator2/1 -> Logical Operator9/1, Logical Operator10/2, Unit Delay Enabled Resettable4/3(Reset), Delay3/1
  Relational Operator3/1 -> Unit Delay Enabled Resettable5/3(Reset), HDL Counter8/1, HDL Counter3/1, signal_edg4/1(In1)
  Relational Operator4/1 -> Logical Operator18/1
  Relational Operator7/1 -> Logical Operator26/1
  Relational Operator8/1 -> Logical Operator29/1, signal_edg6/1(In1)
  Switch1/1 -> Switch13/1
  Switch10/1 -> Relational Operator/1
  Switch11/1 -> Add6/1
  Switch12/1 -> Add2/2
  Switch13/1 -> Add1/2
  Switch14/1 -> Switch3/3
  Switch15/1 -> Add6/2
  Switch16/1 -> [data_wr]
  Switch17/1 -> Compare To Constant24/1, Compare To Constant18/1, Unit Delay Enabled Resettable28/1(data_in), Unit Delay Enabled Resettable15/1(data_in)
  Switch18/1 -> HDL Counter9/3
  Switch2/1 -> Bit Concat/1
  Switch3/1 -> Data Type Conversion10/1
  Switch4/1 -> [count_wr]
  Switch5/1 -> data_mux/1
  Switch6/1 -> Data Type Conversion3/1
  Switch7/1 -> Data Type Conversion11/1
  Switch8/1 -> [addr_wr]
  Switch9/1 -> [RD_BYTE_VAL]
  Unit Delay Enabled Resettable/1(data_out) -> [EN]
  Unit Delay Enabled Resettable1/1(data_out) -> Bit Slice5/1, Bit Slice4/1, Bit Slice3/1
  Unit Delay Enabled Resettable10/1(data_out) -> Out5/1
  Unit Delay Enabled Resettable11/1(data_out) -> Out6/1
  Unit Delay Enabled Resettable12/1(data_out) -> Out7/1
  Unit Delay Enabled Resettable13/1(data_out) -> Out8/1
  Unit Delay Enabled Resettable14/1(data_out) -> [interrypt], irq/1
  Unit Delay Enabled Resettable15/1(data_out) -> [num_wr_byt]
  Unit Delay Enabled Resettable16/1(data_out) -> Delay16/1, signal_edg8/1(In1)
  Unit Delay Enabled Resettable17/1(data_out) -> Index Vector/2
  Unit Delay Enabled Resettable18/1(data_out) -> Index Vector/3
  Unit Delay Enabled Resettable19/1(data_out) -> Index Vector/4
  Unit Delay Enabled Resettable2/1(data_out) -> Compare To Constant21/1
  Unit Delay Enabled Resettable20/1(data_out) -> Index Vector/5
  Unit Delay Enabled Resettable21/1(data_out) -> Index Vector/6
  Unit Delay Enabled Resettable22/1(data_out) -> Index Vector/7
  Unit Delay Enabled Resettable23/1(data_out) -> Index Vector/8
  Unit Delay Enabled Resettable24/1(data_out) -> Index Vector/9
  Unit Delay Enabled Resettable26/1(data_out) -> STATUS/1
  Unit Delay Enabled Resettable28/1(data_out) -> Logical Operator27/1
  Unit Delay Enabled Resettable3/1(data_out) -> Switch3/2, Switch2/2, HDL Counter6/1
  Unit Delay Enabled Resettable4/1(data_out) -> Switch14/2, Switch1/2, HDL Counter7/1
  Unit Delay Enabled Resettable5/1(data_out) -> HDL Counter8/2
  Unit Delay Enabled Resettable6/1(data_out) -> Out1/1
  Unit Delay Enabled Resettable7/1(data_out) -> Out2/1
  Unit Delay Enabled Resettable8/1(data_out) -> Out3/1
  Unit Delay Enabled Resettable9/1(data_out) -> Out4/1
  signal_edg/1(Out1) -> [RD_BYTE]
  signal_edg1/1(Out1) -> Logical Operator20/1, Delay9/1
  signal_edg10/1(Out1) -> [rst_interrypt]
  signal_edg2/1(Out1) -> Logical Operator22/2, Delay11/1, Delay10/1
  signal_edg3/1(Out1) -> HDL Counter10/1
  signal_edg4/1(Out1) -> Delay5/1
  signal_edg5/1(Out1) -> Logical Operator13/2, HDL Counter10/2, [byte_done]
  signal_edg6/1(Out1) -> [write_ok]
  signal_edg7/1(Out1) -> Unit Delay Enabled Resettable16/2(Enb), Unit Delay Enabled Resettable16/1(data_in)
  signal_edg8/1(Out1) -> Logical Operator24/1
  signal_edg9/1(Out1) -> Switch18/2, HDL Counter9/2
